simulink model "Installation_Errors_Sim"  (R2023b)
settings: Solver=FixedStepAuto  StartTime=0.0  StopTime=15  FixedStep=1/10000  RelTol=1e-3
undefined symbols (not defined in the file or in its folder): gyroBias, imuResidualDelay, lpfFreq, lpfZeta, X_num
libraries: Installation_Errors_Lib x7, simulink_extras x2, dspstat3 x1
settings Model: Creator=leoni  LastModifiedBy=leoni

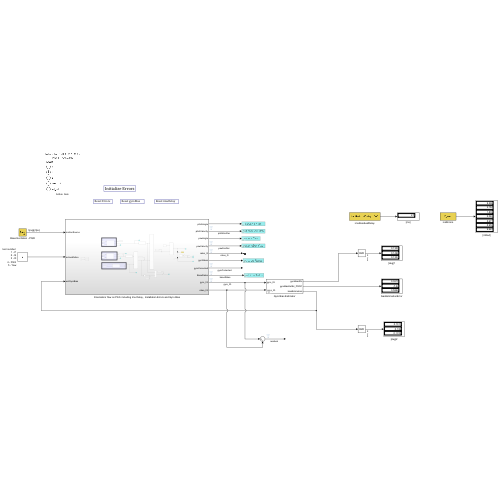
[thumbnail: Simulink's stored preview of the top-level diagram]
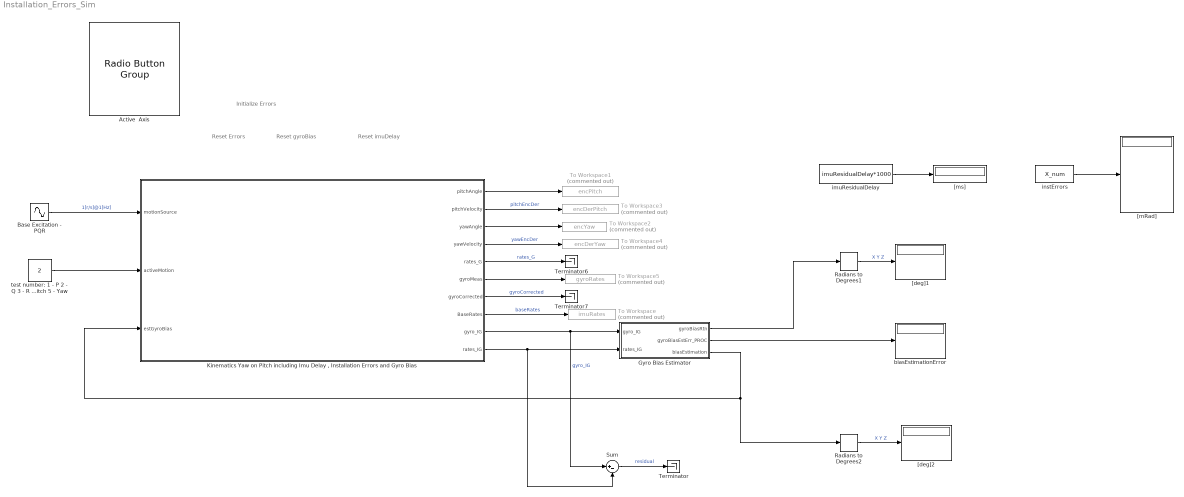
== system Installation_Errors_Sim ==
  note: Reset Errors
  note: Initialize Errors
  note: Reset gyroBias
  note: Reset imuDelay
  Active  Axis : RadioButtonGroup  SelectedLabel=Y  ButtonGroupName=Group
      settings: Values={{'X', 'Y', 'Z', 'theta_dot', 'psi_dot'}, [1 2 3 4 5]}
  Base Excitation - PQR : Sin  Frequency=1*2*pi  SampleTime=0
  Gyro Bias Estimator : Subsystem  mask{lpfFreq=lpfFreq, lpfZeta=lpfZeta}
      mask prompts: lpfFreq "Low Pass Filter Frequency [Hz]"; lpfZeta "Low Pass Filter Zeta"
      mask DialogControl ParameterGroupVar Prompt: LPF Parameters
  "Kinematics Yaw on Pitch including Imu Delay , Installation Errors and Gyro Bias" : Subsystem
  Radians to Degrees1 : simulink_extras/Transformations/Radians to Degrees
  Radians to Degrees2 : simulink_extras/Transformations/Radians to Degrees
  Sum : Sum  Inputs=|+-
  Terminator : Terminator
  Terminator6 : Terminator
  Terminator7 : Terminator
  To Workspace : ToWorkspace  Commented=on  VariableName=imuRates  SaveFormat=Timeseries  SampleTime=-1
  To Workspace1 : ToWorkspace  Commented=on  VariableName=encPitch  SaveFormat=Timeseries  SampleTime=-1
  To Workspace2 : ToWorkspace  Commented=on  VariableName=encYaw  SaveFormat=Timeseries  SampleTime=-1
  To Workspace3 : ToWorkspace  Commented=on  VariableName=encDerPitch  SaveFormat=Timeseries  SampleTime=-1
  To Workspace4 : ToWorkspace  Commented=on  VariableName=encDerYaw  SaveFormat=Timeseries  SampleTime=-1
  To Workspace5 : ToWorkspace  Commented=on  VariableName=gyroRates  SaveFormat=Timeseries  SampleTime=-1
  "[deg]1" : Display
  "[deg]2" : Display
  "[mRad]" : Display
  "[ms]" : Display
  biasEstimationError : Display
  imuResidualDelay : Constant  Value=imuResidualDelay*1000
  instErrors : Constant  Value=X_num
  test number: 1 - P 2 - Q 3 - R 4 - Pitch 5 - Yaw : Constant  Value=2
  wires:
  Base Excitation - PQR/1 -> "Kinematics Yaw on Pitch including Imu Delay , Installation Errors and Gyro Bias"/1(motionSource)  "1[r/s]@1[Hz]"
  test number: 1 - P 2 - Q 3 - R 4 - Pitch 5 - Yaw/1 -> "Kinematics Yaw on Pitch including Imu Delay , Installation Errors and Gyro Bias"/2(activeMotion)
  imuResidualDelay/1 -> "[ms]"/1
  instErrors/1 -> "[mRad]"/1
  Radians to Degrees1/1 -> "[deg]1"/1  "X Y Z"
  "Kinematics Yaw on Pitch including Imu Delay , Installation Errors and Gyro Bias"/1(pitchAngle) -> To Workspace1/1
  "Kinematics Yaw on Pitch including Imu Delay , Installation Errors and Gyro Bias"/2(pitchVelocity) -> To Workspace3/1  "pitchEncDer"
  "Kinematics Yaw on Pitch including Imu Delay , Installation Errors and Gyro Bias"/3(yawAngle) -> To Workspace2/1
  "Kinematics Yaw on Pitch including Imu Delay , Installation Errors and Gyro Bias"/4(yawVelocity) -> To Workspace4/1  "yawEncDer"
  "Kinematics Yaw on Pitch including Imu Delay , Installation Errors and Gyro Bias"/5(rates_G) -> Terminator6/1  "rates_G"
  "Kinematics Yaw on Pitch including Imu Delay , Installation Errors and Gyro Bias"/6(gyroMeas) -> To Workspace5/1
  "Kinematics Yaw on Pitch including Imu Delay , Installation Errors and Gyro Bias"/10(rates_IG) -> Sum/2, Gyro Bias Estimator/2(rates_IG)
  Gyro Bias Estimator/3(biasEstimation) -> "Kinematics Yaw on Pitch including Imu Delay , Installation Errors and Gyro Bias"/3(estGyroBias), Radians to Degrees2/1
  "Kinematics Yaw on Pitch including Imu Delay , Installation Errors and Gyro Bias"/9(gyro_IG) -> Sum/1, Gyro Bias Estimator/1(gyro_IG)  "gyro_IG"
  "Kinematics Yaw on Pitch including Imu Delay , Installation Errors and Gyro Bias"/8(BaseRates) -> To Workspace/1  "baseRates"
  Gyro Bias Estimator/1(gyroBiasRtn) -> Radians to Degrees1/1
  Gyro Bias Estimator/2(gyroBiasEstErr_PROC) -> biasEstimationError/1
  "Kinematics Yaw on Pitch including Imu Delay , Installation Errors and Gyro Bias"/7(gyroCorrected) -> Terminator7/1  "gyroCorrected"
  Radians to Degrees2/1 -> "[deg]2"/1  "X Y Z"
  Sum/1 -> Terminator/1  "residual"

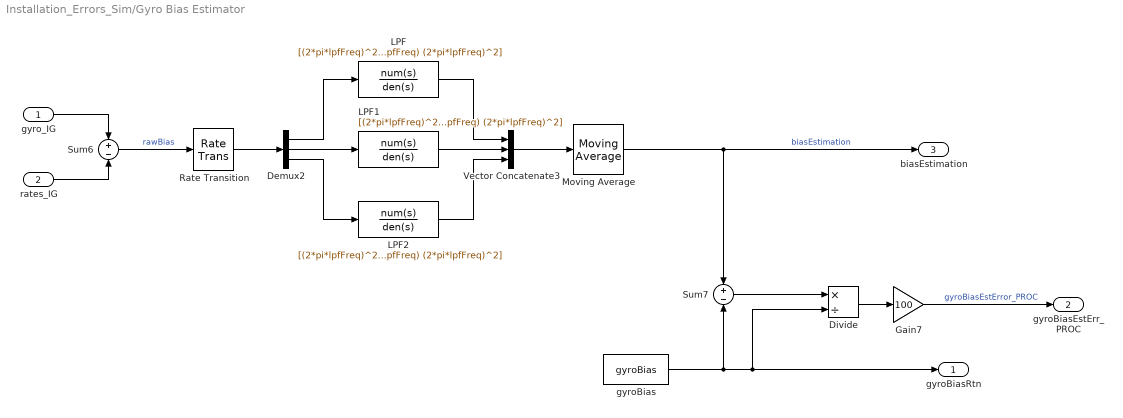
== system Installation_Errors_Sim/Gyro Bias Estimator ==
  gyro_IG : Inport
  rates_IG : Inport  Port=2
  Demux2 : Demux  Outputs=3
  Divide : Product  Inputs=*/
  Gain7 : Gain  Gain=100
  LPF : TransferFcn  Numerator=[(2*pi*lpfFreq)^2]  Denominator=[1 2*lpfZeta*(2*pi*lpfFreq) (2*pi*lpfFreq)^2]
  LPF1 : TransferFcn  Numerator=[(2*pi*lpfFreq)^2]  Denominator=[1 2*lpfZeta*(2*pi*lpfFreq) (2*pi*lpfFreq)^2]
  LPF2 : TransferFcn  Numerator=[(2*pi*lpfFreq)^2]  Denominator=[1 2*lpfZeta*(2*pi*lpfFreq) (2*pi*lpfFreq)^2]
  Moving Average : dspstat3/Moving Average  Method=Exponential weighting  ForgettingFactorPort=off  SpecifyWindowLength=on  WindowLength=4  OverlapLength=3  AllowArbitraryInputLength=off  ForgettingFactor=0.15  SimulateUsing=Code generation
  Rate Transition : RateTransition  OutPortSampleTime=1/2000
  Sum6 : Sum  Inputs=+|-
  Sum7 : Sum  Inputs=+|-
  Vector Concatenate3 : Concatenate  NumInputs=3
  gyroBias : Constant  Value=gyroBias
  gyroBiasRtn : Outport
  gyroBiasEstErr_PROC : Outport  Port=2
  biasEstimation : Outport  Port=3
  wires:
  LPF/1 -> Vector Concatenate3/1
  Vector Concatenate3/1 -> Moving Average/1
  Sum6/1 -> Rate Transition/1  "rawBias"
  rates_IG/1 -> Sum6/2
  Moving Average/1 -> Sum7/1, biasEstimation/1  "biasEstimation"
  LPF1/1 -> Vector Concatenate3/2
  gyro_IG/1 -> Sum6/1
  Demux2/3 -> LPF2/1
  Demux2/2 -> LPF1/1
  Demux2/1 -> LPF/1
  Rate Transition/1 -> Demux2/1
  LPF2/1 -> Vector Concatenate3/3
  Divide/1 -> Gain7/1
  gyroBias/1 -> gyroBiasRtn/1, Divide/2, Sum7/2
  Gain7/1 -> gyroBiasEstErr_PROC/1  "gyroBiasEstError_PROC"
  Sum7/1 -> Divide/1

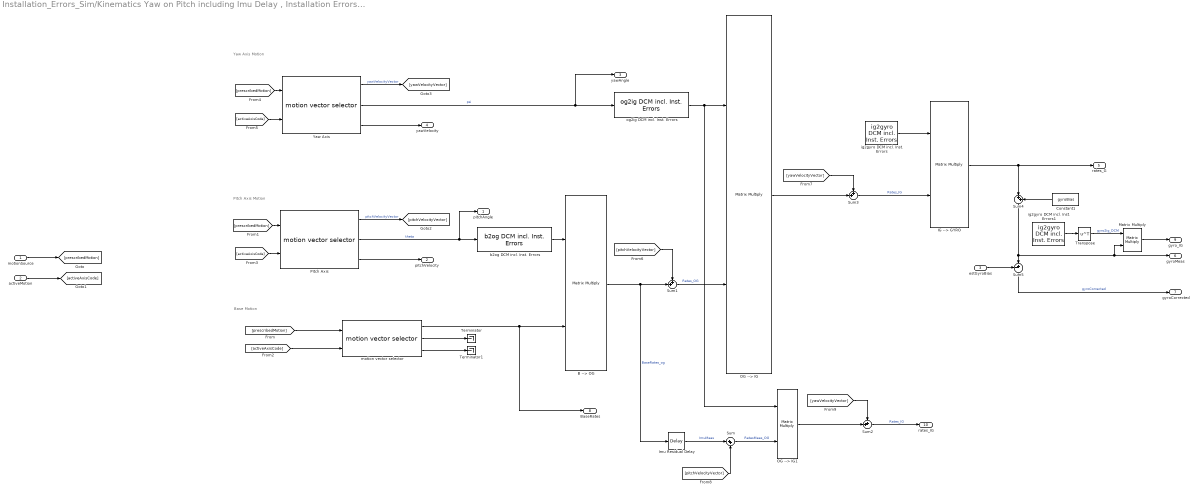
== system Installation_Errors_Sim/Kinematics Yaw on Pitch including Imu Delay , Installation Errors and Gyro Bias ==
  note: Base Motion
  note: Yaw Axis Motion
  note: Pitch Axis Motion
  motionSource : Inport
  activeMotion : Inport  Port=2
  estGyroBias : Inport  Port=3
  B --> OG : Product  Multiplication=Matrix(*)
  Constant1 : Constant  Value=gyroBias
  IG --> GYRO : Product  Multiplication=Matrix(*)
  Imu Residual Delay : TransportDelay  DelayTime=imuResidualDelay
  Matrix Multiply : Product  Multiplication=Matrix(*)
  OG --> IG : Product  Multiplication=Matrix(*)
  OG --> IG1 : Product  Multiplication=Matrix(*)
  Pitch Axis : Installation_Errors_Lib/motion vector selector  SystemSampleTime=-1  VariantActivationTime=update diagram  AllowFlexibleInterface=on  Latency=0  AutoFrameSizeCalculation=off
      link override Vx: axisCode=None
      link override Vz: axisCode=None
  Sum : Sum  Inputs=|++
  Sum1 : Sum  Inputs=++|
  Sum2 : Sum  Inputs=++|
  Sum3 : Sum  Inputs=++|
  Sum4 : Sum  Inputs=|++
  Sum5 : Sum  Inputs=-+|
  Terminator : Terminator
  Terminator1 : Terminator
  Transpose : Math  Operator=transpose
  Yaw Axis : Installation_Errors_Lib/motion vector selector  SystemSampleTime=-1  VariantActivationTime=update diagram  AllowFlexibleInterface=on  Latency=0  AutoFrameSizeCalculation=off
      link override Vx: axisCode=None
      link override Vy: axisCode=None
      link override Vz: axisCode=Yaw
  b2og DCM incl. Inst. Errors : Installation_Errors_Lib/b2og DCM incl. Inst. Errors  eoa1=X_num(1)  eoa3=X_num(2)  theta_o=X_num(6)
  ig2gyro DCM incl. Inst. Errors : Installation_Errors_Lib/ig2gyro DCM incl. Inst. Errors  eg1=X_num(4)  eg2=X_num(5)
  ig2gyro DCM incl. Inst. Errors1 : Installation_Errors_Lib/ig2gyro DCM incl. Inst. Errors  eg1=X_num(4)  eg2=X_num(5)
  motion vector selector : Installation_Errors_Lib/motion vector selector  SystemSampleTime=-1  VariantActivationTime=update diagram  AllowFlexibleInterface=on  Latency=0  AutoFrameSizeCalculation=off
      link override Vx: axisCode=P
      link override Vy: axisCode=Q
      link override Vz: axisCode=R
  og2ig DCM incl. Inst. Errors : Installation_Errors_Lib/og2ig DCM incl. Inst. Errors  eia1=X_num(3)  psi_o=X_num(7)
  pitchAngle : Outport
  pitchVelocity : Outport  Port=2
  yawAngle : Outport  Port=3
  yawVelocity : Outport  Port=4
  rates_G : Outport  Port=5
  gyroMeas : Outport  Port=6
  gyroCorrected : Outport  Port=7
  BaseRates : Outport  Port=8
  gyro_IG : Outport  Port=9
  rates_IG : Outport  Port=10
  wires:
  Sum4/1 -> Sum5/2, Matrix Multiply/2, gyroMeas/1
  B --> OG/1 -> Sum1/2, Imu Residual Delay/1  "BaseRates_og"
  Imu Residual Delay/1 -> Sum/1  "ImuMeas"
  activeMotion/1 -> [activeAxisCode]
  Sum3/1 -> IG --> GYRO/2  "Rates_IG"
  Pitch Axis/2 -> pitchAngle/1, b2og DCM incl. Inst. Errors/1  "theta"
  Sum5/1 -> gyroCorrected/1  "gyroCorrected"
  Sum1/1 -> OG --> IG/2  "Rates_OG"
  Constant1/1 -> Sum4/2
  OG --> IG/1 -> Sum3/2
  motionSource/1 -> [prescribedMotion]
  Yaw Axis/2 -> og2ig DCM incl. Inst. Errors/1, yawAngle/1  "psi"
  estGyroBias/1 -> Sum5/1
  b2og DCM incl. Inst. Errors/1 -> B --> OG/1
  og2ig DCM incl. Inst. Errors/1 -> OG --> IG1/1, OG --> IG/1
  ig2gyro DCM incl. Inst. Errors/1 -> IG --> GYRO/1
  IG --> GYRO/1 -> Sum4/1, rates_G/1
  [prescribedMotion] -> Pitch Axis/1
  [activeAxisCode] -> Pitch Axis/2
  [activeAxisCode] -> Yaw Axis/2
  [prescribedMotion] -> Yaw Axis/1
  motion vector selector/1 -> BaseRates/1, B --> OG/2
  motion vector selector/2 -> Terminator/1
  motion vector selector/3 -> Terminator1/1
  [activeAxisCode] -> motion vector selector/2
  [prescribedMotion] -> motion vector selector/1
  Pitch Axis/3 -> pitchVelocity/1
  Pitch Axis/1 -> [pitchVelocityVector]  "pitchVelocityVector"
  Yaw Axis/3 -> yawVelocity/1
  [pitchVelocityVector] -> Sum1/1
  Yaw Axis/1 -> [yawVelocityVector]  "yawVelocityVector"
  [yawVelocityVector] -> Sum3/1
  [pitchVelocityVector] -> Sum/2
  Sum/1 -> OG --> IG1/2  "RatesMeas_OG"
  [yawVelocityVector] -> Sum2/1
  OG --> IG1/1 -> Sum2/2
  Sum2/1 -> rates_IG/1  "Rates_IG"
  ig2gyro DCM incl. Inst. Errors1/1 -> Transpose/1
  Matrix Multiply/1 -> gyro_IG/1
  Transpose/1 -> Matrix Multiply/1  "gyro2ig_DCM"
